simulink model "VOO_ONLY"  (R2022b)
settings: Solver=FixedStepAuto  StartTime=0.0  StopTime=10.0  FixedStep=1e-3  RelTol=1e-3  EnableMultiTasking=on
undefined symbols (not defined in the file): D10, D11, D12, D2, D5, D8, D9, PTA0, PTA2, PTB9, PTC4, PTD0, PTD2, PTD3
libraries: frdmk64flib x7
settings Model: ExtModeTrigDuration=5  Creator=aldenluscher  LastModifiedBy=andre
settings OptimizationCC: EnhancedBackFolding=on  PassReuseOutputArgsAs=Individual arguments  ZeroExternalMemoryAtStartup=off  ZeroInternalMemoryAtStartup=off  MaxStackSize=64  OptimizeBlockOrder=speed  DifferentSizesBufferReuse=on  OptimizationCustomize=off  EfficientTunableParamExpr=on
settings DebuggingCC: ParameterTunabilityLossMsg=error
settings HardwareCC: ProdBitPerPointer=32  ProdBitPerSizeT=32  ProdBitPerPtrDiffT=32  ProdLargestAtomicInteger=Long  ProdLargestAtomicFloat=Double  ProdWordSize=32  ProdHWDeviceType=ARM Compatible->ARM Cortex
settings SFSimCC: MATLABDynamicMemAlloc=off
settings RTWCC: Description=Embedded Coder  SystemTargetFile=ert.tlc  HardwareBoard=NXP FRDM-K64F  TLCOptions="-aInlineSetEventsForThisBaseRateFcn=TLC_FALSE -aSuppressMultiTaskScheduler=TLC_FALSE  -aRateBasedStepFcn=0"  TemplateMakefile=ert_default_tmf  Toolchain=GNU Tools for ARM Embedded Processors
settings CodeAppCC: ForceParamTrailComments=on  IgnoreCustomStorageClasses=off  OperatorAnnotations=on  SimulinkDataObjDesc=on  SFDataObjDesc=on  InsertBlockDesc=on
settings ERTTargetCC: ExtModeTransport=4  ExtModeMexFile=sendToCommService

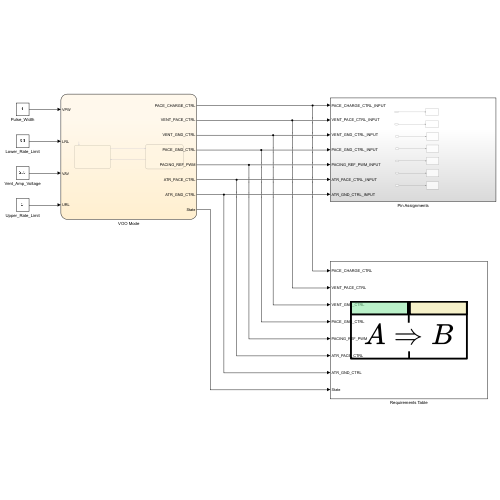
[thumbnail: Simulink's stored preview of the top-level diagram]
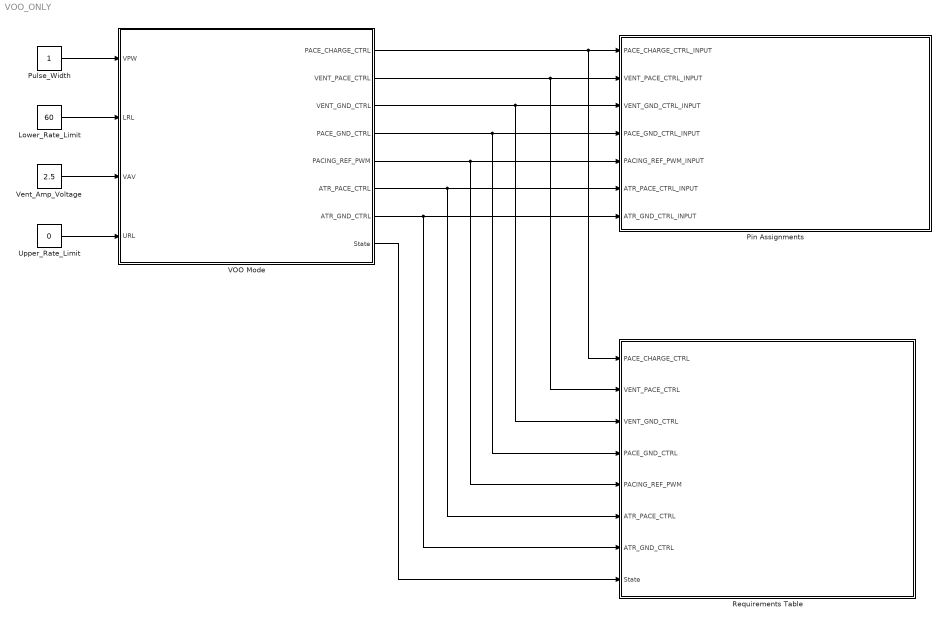
== system VOO_ONLY ==
  Lower_Rate_Limit : Constant  Value=60
  Pin Assignments : Subsystem
  Pulse_Width : Constant
  Requirements Table : Requirements Table  TreatAsAtomicUnit=on
  Upper_Rate_Limit : Constant  Value=0
  VOO Mode : Stateflow chart  TreatAsAtomicUnit=on
      settings: PortSchema="{\"entries\":[{\"content\":{\"sides\":[{\"content\":{\"connectorIds\":[\"In1\",\"In2\",\"In3\",\"In4\"]},\"type\":\"ConnectorPlacement.EquallySpacedRectSide\",\"uuid\":\"ab30f6e3-f4a9-4bd5-815e-4ef92b766934\"},{\"content\":{\"connectorIds\":[\"Out1\",\"Out4\",\"Out3\",\"Out2\",\"Out5\",\"Out6\",\"Out7\",\"Out8\"],\"side\":\"RIGHT\"},\"type\":\"ConnectorPlacement.EquallySpacedRectSide\",\"uuid\":\"1d0d5e4f-590d-4361-90fd-546c5207ab80\"},{\"content\":{\"connectorIds\":[],\"side\":\"TOP\"},\"type\":\"ConnectorPlacement.EquallySpacedRectSide\",\"uuid\":\"49517801-e549-4c52-be80-c1c6727c26aa\"},{\"content\":{\"connectorIds\":[],\"side\":\"BOTTOM\"},\"type\":\"ConnectorPlacement.EquallySpacedRectSide\",\"uuid\":\"3a20310d-7367-4e60-a663-7e5c4f14e519\"}]},\"type\":\"ConnectorPlacement.EquallySpacedConnector\",\"uuid\":\"1ff6ee75-2732-4076-aa82-0b614a2ae219\"}],\"packageUris\":[\"http://schema.mathworks.com/mf0/Connector/R2020b\"],\"version\":\"1.0\"}"
  Vent_Amp_Voltage : Constant  Value=2.5
  wires:
  VOO Mode/5(PACING_REF_PWM) -> Requirements Table/5(PACING_REF_PWM), Pin Assignments/5(PACING_REF_PWM_INPUT)
  VOO Mode/4(VENT_PACE_CTRL) -> Requirements Table/2(VENT_PACE_CTRL), Pin Assignments/2(VENT_PACE_CTRL_INPUT)
  VOO Mode/3(VENT_GND_CTRL) -> Requirements Table/3(VENT_GND_CTRL), Pin Assignments/3(VENT_GND_CTRL_INPUT)
  VOO Mode/2(PACE_GND_CTRL) -> Requirements Table/4(PACE_GND_CTRL), Pin Assignments/4(PACE_GND_CTRL_INPUT)
  VOO Mode/1(PACE_CHARGE_CTRL) -> Requirements Table/1(PACE_CHARGE_CTRL), Pin Assignments/1(PACE_CHARGE_CTRL_INPUT)
  Pulse_Width/1 -> VOO Mode/1(VPW)
  Vent_Amp_Voltage/1 -> VOO Mode/3(VAV)
  Lower_Rate_Limit/1 -> VOO Mode/2(LRL)
  Upper_Rate_Limit/1 -> VOO Mode/4(URL)
  VOO Mode/8(State) -> Requirements Table/8(State)
  VOO Mode/6(ATR_PACE_CTRL) -> Pin Assignments/6(ATR_PACE_CTRL_INPUT), Requirements Table/6(ATR_PACE_CTRL)
  VOO Mode/7(ATR_GND_CTRL) -> Pin Assignments/7(ATR_GND_CTRL_INPUT), Requirements Table/7(ATR_GND_CTRL)

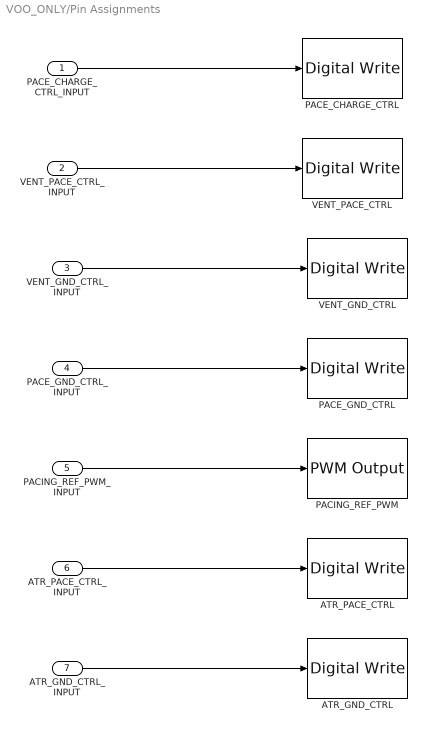
== system VOO_ONLY/Pin Assignments ==
  PACE_CHARGE_CTRL_INPUT : Inport
  VENT_PACE_CTRL_INPUT : Inport  Port=2
  VENT_GND_CTRL_INPUT : Inport  Port=3
  PACE_GND_CTRL_INPUT : Inport  Port=4
  PACING_REF_PWM_INPUT : Inport  Port=5
  ATR_PACE_CTRL_INPUT : Inport  Port=6
  ATR_GND_CTRL_INPUT : Inport  Port=7
  ATR_GND_CTRL : frdmk64flib/Digital Write  Whichpin=PTD2 (D11)
  ATR_PACE_CTRL : frdmk64flib/Digital Write  Whichpin=PTA0 (D8)
  PACE_CHARGE_CTRL : frdmk64flib/Digital Write  Whichpin=PTB9 (D2)
  PACE_GND_CTRL : frdmk64flib/Digital Write  Whichpin=PTD0 (D10)
  PACING_REF_PWM : frdmk64flib/PWM Output  Whichpin=PTA2 (D5)  InitialFrequency=2000  InitialDutyCycle=0
  VENT_GND_CTRL : frdmk64flib/Digital Write  Whichpin=PTD3 (D12)
  VENT_PACE_CTRL : frdmk64flib/Digital Write  Whichpin=PTC4 (D9)
  wires:
  VENT_PACE_CTRL_INPUT/1 -> VENT_PACE_CTRL/1
  PACE_GND_CTRL_INPUT/1 -> PACE_GND_CTRL/1
  PACE_CHARGE_CTRL_INPUT/1 -> PACE_CHARGE_CTRL/1
  PACING_REF_PWM_INPUT/1 -> PACING_REF_PWM/1
  VENT_GND_CTRL_INPUT/1 -> VENT_GND_CTRL/1
  ATR_PACE_CTRL_INPUT/1 -> ATR_PACE_CTRL/1
  ATR_GND_CTRL_INPUT/1 -> ATR_GND_CTRL/1

== stateflow chart VOO_ONLY/Requirements Table ==
  (default) -> (junction 1073742518)
  (junction 1073742518) -> (junction 1073742519) : {
      | % SF_REQ_REV_07
      | }
  (junction 1073742519) -> (junction 1073742521) : {
      | % HEADER_ASSIGNMENTS
      |
      | }
  (junction 1073742521) -> (junction 1073742523) : {
      | % START_A_4
      | }
  (junction 1073742523) -> (junction 1073742525) : {
      | }
  (junction 1073742525) -> (junction 1073742527)
  (junction 1073742527) -> (junction 1073742529) : {
      | }
  (junction 1073742529) -> (junction 1073742531) : {
      | % END_A_4
      | }
  (junction 1073742531) -> (junction 1073742533) : {
      | % START_R_1
      | }
  (junction 1073742533) -> (junction 1073742535) : {
      | }
  (junction 1073742535) -> (junction 1073742537)
  (junction 1073742537) -> (junction 1073742539) [order 1] : [(((State) == (0)))]
  (junction 1073742537) -> (junction 1073742545) [order 2]
  (junction 1073742539) -> (junction 1073742541) : {
      | reqtable_postcondition((((PACE_CHARGE_CTRL) == (1))) && (((PACE_GND_CTRL) == (1))) && (((VENT_PACE_CTRL) == (0))) && (((VENT_GND_CTRL) == (1))) && (((ATR_PACE_CTRL) == (0))) && (((ATR_GND_CTRL) == (0))) && (0<=PACING_REF_PWM<=100), 'R:1');
      |
      |
      | }
  (junction 1073742541) -> (junction 1073742543) : {
      | }
  (junction 1073742543) -> (junction 1073742545)
  (junction 1073742545) -> (junction 1073742547)
  (junction 1073742547) -> (junction 1073742549) : {
      | % END_R_1
      | }
  (junction 1073742549) -> (junction 1073742551) : {
      | % START_R_7
      | }
  (junction 1073742551) -> (junction 1073742553) : {
      | }
  (junction 1073742553) -> (junction 1073742555)
  (junction 1073742555) -> (junction 1073742557) [order 1] : [(((State) == (1)))]
  (junction 1073742555) -> (junction 1073742563) [order 2]
  (junction 1073742557) -> (junction 1073742559) : {
      | reqtable_postcondition((((PACE_CHARGE_CTRL) == (0))) && (((PACE_GND_CTRL) == (1))) && (((VENT_PACE_CTRL) == (1))) && (((VENT_GND_CTRL) == (0))) && (((ATR_PACE_CTRL) == (0))) && (((ATR_GND_CTRL) == (0))), 'R:2');
      |
      |
      | }
  (junction 1073742559) -> (junction 1073742561) : {
      | }
  (junction 1073742561) -> (junction 1073742563)
  (junction 1073742563) -> (junction 1073742565)
  (junction 1073742565) -> (junction 1073742567) : {
      | % END_R_7
      | }
  data: PACE_CHARGE_CTRL input; VENT_PACE_CTRL input; VENT_GND_CTRL input; PACE_GND_CTRL input; PACING_REF_PWM input; ATR_PACE_CTRL input; ATR_GND_CTRL input; State input

== stateflow chart VOO_ONLY/VOO Mode ==
  state Pacing_
    PACE_CHARGE_CTRL = 0;
    PACE_GND_CTRL = 1;
    VENT_GND_CTRL = 0;
    VENT_PACE_CTRL = 1;
    ATR_PACE_CTRL = 0;
    ATR_GND_CTRL = 0;
    State = 1;
  state Charging_
    PACING_REF_PWM = 100*(VAV/5);
    PACING_PERIOD = (60000/LRL);
    PACE_CHARGE_CTRL = 1;
    PACE_GND_CTRL = 1;
    VENT_GND_CTRL = 1;
    VENT_PACE_CTRL = 0;
    ATR_PACE_CTRL = 0;
    ATR_GND_CTRL = 0;
    State = 0;
  note: Charging time = Full length of period - pulse width
  note: Pacing time = Ventricle pulse width
  note: VAV is the ventricle amplitude
      | LRL is the lower rate limit
  (default) -> Charging_
  Charging_ -> Pacing_ : after(PACING_PERIOD-VPW,msec)
  Pacing_ -> Charging_ : after(VPW,msec)
  data: PACE_CHARGE_CTRL output; PACE_GND_CTRL output; VENT_GND_CTRL output; VENT_PACE_CTRL output; PACING_REF_PWM output; VPW input; LRL input; VAV input; PACING_PERIOD local; URL input; ATR_PACE_CTRL output; ATR_GND_CTRL output; State output int8 [0..1] =int8(0)
